simulink model "modelNEWw"  (R2022a)
settings: Solver=VariableStepAuto  StartTime=0.0  StopTime=60  RelTol=1e-3
settings Model: Creator=Angela  LastModifiedBy=Angela

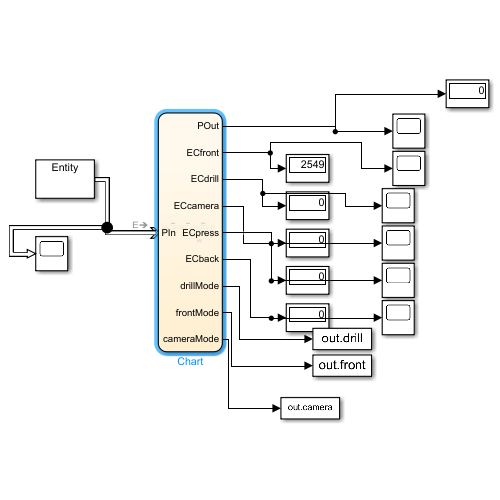
[thumbnail: Simulink's stored preview of the top-level diagram]
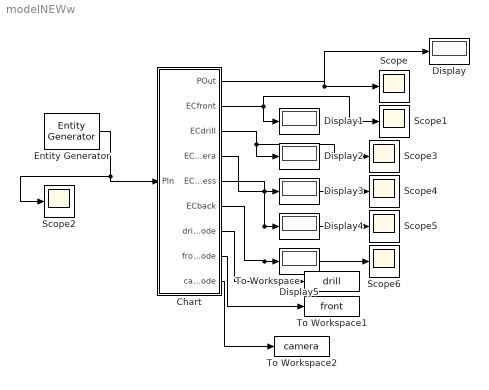
== system modelNEWw ==
  Chart : Stateflow chart  TreatAsAtomicUnit=on
  Display{,1..5} (6 alike) : Display
  Entity Generator : EntityGenerator  OutputPortMessageModes=m  Period=5  GenerateEntityAtSimulationStart=off  EntityType=Structured  EntityTypeName=Entity
  Scope{,1..6} (7 alike) : Scope
  To Workspace : ToWorkspace  VariableName=drill  SaveFormat=Timeseries  SampleTime=-1
  To Workspace1 : ToWorkspace  VariableName=front  SaveFormat=Timeseries  SampleTime=-1
  To Workspace2 : ToWorkspace  VariableName=camera  SaveFormat=Timeseries  SampleTime=-1
  wires:
  Entity Generator/1 -> Scope2/1, Chart/1(PIn)
  Chart/1(POut) -> Display/1, Scope/1
  Chart/2(ECfront) -> Display1/1, Scope1/1
  Chart/3(ECdrill) -> Display2/1, Scope3/1
  Chart/4(ECcamera) -> Scope4/1, Display3/1
  Chart/5(ECpress) -> Scope5/1, Display4/1
  Chart/6(ECback) -> Scope6/1, Display5/1
  Chart/7(" drillMode") -> To Workspace/1
  Chart/8(" frontMode") -> To Workspace1/1
  Chart/9(" cameraMode") -> To Workspace2/1

== stateflow chart modelNEWw/Chart ==
  settings: sampleTime=0
  state back [parallel]
    settings: executionOrder=4
    state Idle
      entry:
      processing=0;
    state Working
      entry:
      processing=1;
      exit:
      ECback=eFront(0,CTback)+ECback;
      Counter=Counter+1
    (default) -> back.Idle
    back.Idle -> back.Working : Pin{press.queue=press.queue-1}
    back.Working -> back.Idle : after(CTback,sec){queue=queue+1}/{POut=POut+1}
  state press [parallel]
    settings: executionOrder=3
    state Idle
      entry:
      processing=0;
    state Working
      entry:
      processing=1;
      exit:
      ECpress=ePress(0,CTpress)+ECpress;
      Counter=Counter+1
    (default) -> press.Idle
    press.Idle -> press.Working : Pin{camera.queue=camera.queue-1}
    press.Working -> press.Idle : after(CTpress,sec){queue=queue+1}/{back.Pin}
  state camera [parallel]
    settings: executionOrder=2
    state Idle
      entry:
      processing=0;
    state Working
      entry:
      processing=1;
      exit:
      ECcamera=eCamera(0,CTcamera)+ECcamera;
      Counter=Counter+1
    (default) -> camera.Idle
    camera.Idle -> camera.Working : Pin{drill.queue=drill.queue-1}
    camera.Working -> camera.Idle : after(CTcamera,sec){queue=queue+1}/{press.Pin}
  state drill [parallel]
    settings: executionOrder=1
    state Idle
      entry:
      processing=0;
    state Working
      entry:
      processing=1;
      exit:
      ECdrill=eDrill(0,CTdrill)+ECdrill;
      Counter=Counter+1
    (default) -> drill.Idle
    drill.Idle -> drill.Working : Pin{front.queue=front.queue-1}
    drill.Working -> drill.Idle : after(CTdrill,sec){queue=queue+1}/{camera.Pin}
  state front [parallel]
    settings: executionOrder=5
    state Working
      entry:
      processing=1;
      exit:
      ECfront=ePress(0,CTfront)+ECfront;
      Counter=Counter+1
    state Idle
      entry:
      processing=0;
    (default) -> front.Idle
    front.Idle -> front.Working : PIn
    front.Working -> front.Idle : after(CTfront,sec){queue=queue+1}/{drill.Pin}
  data: a function_input; b function_input; y function_output; a function_input; b function_input; y function_output; a function_input; b function_input; y function_output; processing local =0; CTback constant double =15; Counter local double =0; queue local double =0; processing local =0; CTpress constant double =15; Counter local double =0; queue local double =0; processing local =0; CTcamera constant double =15; Counter local double =0; queue local double =0; processing local =0; CTdrill constant double =50; Counter local double =0; queue local double =0; processing local =0; CTfront constant double =10; Counter local double =0; queue local =0; a function_input; b function_input; y function_output; POut output =0; ECfront output =0; ECdrill output =0; ECcamera output =0; PIn input; ECpress output =0; ECback output =0; drillMode output Enum: drillModeType; frontMode output Enum: frontModeType; cameraMode output Enum: cameraModeType
  events: Pin local FUNCTION_CALL_EVENT; Pin local FUNCTION_CALL_EVENT; Pin local FUNCTION_CALL_EVENT; Pin local FUNCTION_CALL_EVENT
  function y = eFront(a,b):
    | function y = eFront(a,b)
    | y=integral(@(x) -0.000516*x.^4+0.0277*x.^3-0.473*x.^2+2.77*x+47,a,b);
    | end
  function y = ePress(a,b):
    | function y = ePress(a,b)
    | y=integral(@(x) -0.000516*x.^4+0.0277*x.^3-0.473*x.^2+2.77*x+47,a,b);
    | end
  function y = eCamera(a,b):
    | function y = eCamera(a,b)
    | y=integral(@(x) -0.000516*x.^4+0.0277*x.^3-0.473*x.^2+2.77*x+47,a,b);
    | end
  function y = eDrill(a,b):
    | function y = eDrill(a,b)
    | y=integral(@(x) -0.000516*x.^4+0.0277*x.^3-0.473*x.^2+2.77*x+47,a,b);
    | end
